simulink library "AtomicLibrary"
PostLoadFcn:
  | PacketBusGenerator; RailCabBusGenerator
(part 5 of 8)

== stateflow chart Master_Slave_Assignment_comp ==
  state chart
    state chartRegion [parallel]
      state Main
        state Synchronization [parallel]
          state Sleep
            entry: clientAvailableStatechart = true
            exit: clientAvailableStatechart = false
          state State
            entry: clientAvailableStatechart = true; masterAvailableStatechart = true
            exit: clientAvailableStatechart = false; masterAvailableStatechart = false
          state Client
          state Master
          state End
            entry: clientAvailableStatechart = true; masterAvailableStatechart = true
            exit: clientAvailableStatechart = false; masterAvailableStatechart = false
          chart.chartRegion.Main.Synchronization.Client -> End
          Master -> End
          Sleep -> chart.chartRegion.Main.Synchronization.Client : client
          State -> chart.chartRegion.Main.Synchronization.Client [order 2] : client
          End -> chart.chartRegion.Main.Synchronization.Client [order 1] : client
          State -> Master [order 1] : master
          End -> Master [order 2] : master
        state Master_Slave_Ass_Competitor [parallel]
          state Unset
            entry: startAssignmentAvailableMaster_Slave_Assignment_Competitor = true
            exit: startAssignmentAvailableMaster_Slave_Assignment_Competitor = false
          state MasterRequest
            entry: reset(c0)
          state MasterOk
          state Client
          state Inv_Error
          Unset -> chart.chartRegion.Main.Master_Slave_Ass_Competitor.Client [order 1]
          MasterRequest -> Unset [order 1] : [time(c0) > 20]
          MasterOk -> Unset
          Unset -> MasterRequest [order 2] : startAssignment
          MasterRequest -> Inv_Error [order 3] : [time(c0) > 20]
    state DataInit [parallel]
    DataInit -> DataInit
  (default) -> Sleep
  (default) -> Unset
  (default) -> Main
  (default) -> chart
  data: c0 local double =0.0; clientAvailableStatechart local boolean =false; masterAvailableStatechart local boolean =false; startAssignmentAvailableMaster_Slave_Assignment_Competitor local boolean =false; evtQueueIn function_input; param function_input; paramQueueIn function_input; event function_input; evtQueue function_output; paramQueue function_output; event function_input; evtQueue function_input; available function_output; event function_input; evtQueueIn function_input; paramQueueIn function_input; evtQueue function_output; paramQueue function_output; parameter function_output; clock function_input; logicalTime function_output; clock function_input
  events: startAssignment local EITHER_EDGE_EVENT; client local EITHER_EDGE_EVENT; master local EITHER_EDGE_EVENT
  function enqueue:
    | function [evtQueue, paramQueue] = enqueue(event, evtQueueIn, param, paramQueueIn) %eml 
    |  evtQueue = evtQueueIn; 
    |  paramQueue = paramQueueIn; 
    |  for i = 1:length(evtQueueIn) 
    |  if evtQueueIn(i) == uint8(0) 
    |  evtQueueIn(i) = event; 
    |  paramQueue(i) = param; 
    |  return 
    |  end 
    |  end
  function checkQueue:
    | function available = checkQueue(event, evtQueue) %eml 
    |  available = false; 
    |  for i = 1:length(evtQueue) 
    |      if evtQueue(i) == event 
    |          available = true;    
    |          return 
    |      end 
    |  end
  function dequeue:
    | function [evtQueue, paramQueue, parameter] = dequeue(event, evtQueueIn, paramQueueIn) %eml 
    |  evtQueue = evtQueueIn; 
    |  paramQueue = paramQueueIn; 
    |  parameter = 0; 
    |  for i = 1:length(evtQueue) 
    |  if evtQueue(i) == event 
    |  parameter = paramQueue(i); 
    |  for j = i:length(evtQueue)-1 
    |   evtQueue(j) = evtQueue(j+1); 
    |  paramQueue(j) = paramQueue(j+1); 
    |  end 
    |  evtQueue(length(evtQueue)) = 0; 
    |  paramQueue(length(paramQueue)) = 0; 
    |  return 
    |  end 
    |  end
  function time:
    | function logicalTime = time(clock) 
    |  sample = 0.01;  % the sample time of the system clock 
    |  %convert to pass units of time after last reset 
    |  logicalTime = uint32((clockSignal - clock)/sample);
  function reset:
    | function reset(clock) 
    |  %set clock variable to current time 
    |  clock = clockSignal;

== stateflow chart TestTurnTransmission/TestTurnTransmission_Statechart ==
  state chart
    state chartRegion [parallel]
      state Main
        state synchronization [parallel]
          state MyTurn
          state Initial
            entry: turnCHAvailableStatechart = true
            exit: turnCHAvailableStatechart = false
          state YourTurn
            entry: turnCHAvailableStatechart = true
            exit: turnCHAvailableStatechart = false
          Initial -> chart.chartRegion.Main.synchronization.MyTurn [order 2] : turnCH
          chart.chartRegion.Main.synchronization.YourTurn -> chart.chartRegion.Main.synchronization.MyTurn : turnCH
          chart.chartRegion.Main.synchronization.MyTurn -> chart.chartRegion.Main.synchronization.YourTurn : [turnCHAvailableTurn_transmission_partner]{send(turnCH, turn_transmission_partner)}
          Initial -> chart.chartRegion.Main.synchronization.YourTurn [order 1] : [turnCHAvailableTurn_transmission_partner]{send(turnCH, turn_transmission_partner)}
        state turn_transmission_partner [parallel]
          state Inactive
            entry: turnCHAvailableTurn_Transmission_Partner = true
            exit: turnCHAvailableTurn_Transmission_Partner = false
          state TimeOut
          state MyTurn
            entry: turnCHAvailableTurn_Transmission_Partner = true
            exit: turnCHAvailableTurn_Transmission_Partner = false
          state YourTurn
          state Inv_Error
          TimeOut -> Inactive
          chart.chartRegion.Main.turn_transmission_partner.MyTurn -> Inactive [order 2]
          chart.chartRegion.Main.turn_transmission_partner.MyTurn -> TimeOut [order 3] : [time(c0) > 20]
          chart.chartRegion.Main.turn_transmission_partner.YourTurn -> Inactive [order 3]
          chart.chartRegion.Main.turn_transmission_partner.YourTurn -> TimeOut [order 2] : [time(c0) > 20]
          Inactive -> chart.chartRegion.Main.turn_transmission_partner.YourTurn [order 1] : turnCH{[turn_transmission_partnerEvtWriteOut, turn_transmission_partnerParamWriteOut] = enqueue(EVT_TURN, turn_transmission_partnerEvtWriteOut, turn_transmission_partnerParamWriteOut)}
          chart.chartRegion.Main.turn_transmission_partner.MyTurn -> chart.chartRegion.Main.turn_transmission_partner.YourTurn [order 1] : turnCH{[turn_transmission_partnerEvtWriteOut, turn_transmission_partnerParamWriteOut] = enqueue(EVT_TURN, turn_transmission_partnerEvtWriteOut, turn_transmission_partnerParamWriteOut)}
          chart.chartRegion.Main.turn_transmission_partner.YourTurn -> chart.chartRegion.Main.turn_transmission_partner.MyTurn [order 3] : [(turnCHAvailableSynchronization) && ([checkQueue(EVT_TURN, turn_transmission_partnerEvtReadOut)])]{send(turnCH, synchronization)}
          Inactive -> chart.chartRegion.Main.turn_transmission_partner.MyTurn [order 3] : [(turnCHAvailableSynchronization) && ([checkQueue(EVT_TURN, turn_transmission_partnerEvtReadOut)])]{send(turnCH, synchronization)}
          chart.chartRegion.Main.turn_transmission_partner.MyTurn -> Inv_Error [order 4] : [time(c0) > 20]
          chart.chartRegion.Main.turn_transmission_partner.YourTurn -> Inv_Error [order 4] : [time(c0) > 20]
    state DataInit [parallel]
    DataInit -> DataInit : {turn_transmission_partnerEvtWriteOut = turn_transmission_partnerEvtWriteIn;
        | turn_transmission_partnerParamWriteOut = turn_transmission_partnerParamWriteIn;
        | turn_transmission_partnerEvtReadOut = turn_transmission_partnerEvtReadIn;
        | turn_transmission_partnerParamReadOut = turn_transmission_partnerParamReadIn;
        | }
  (default) -> Initial
  (default) -> Inactive
  (default) -> Main
  (default) -> chart
  data: EVT_TURN constant uint32 =7; c0 local double =0.0; EVT_TURN constant uint32 =7; turnCHAvailableStatechart local boolean =false; turnCHAvailableTurn_Transmission_Partner local boolean =false; evtQueueIn function_input; param function_input; paramQueueIn function_input; event function_input; evtQueue function_output; paramQueue function_output; event function_input; evtQueue function_input; available function_output; event function_input; evtQueueIn function_input; paramQueueIn function_input; evtQueue function_output; paramQueue function_output; parameter function_output; clock function_input; logicalTime function_output; clock function_input; clockSignal input; turn_transmission_partnerReadIn input; turn_transmission_partnerParamReadIn input; turn_transmission_partnerWriteIn input; turn_transmission_partnerParamWriteIn input; turn_transmission_partnerReadOut output; turn_transmission_partnerParamReadOut output; turn_transmission_partnerWriteOut output; turn_transmission_partnerParamWriteOut output
  events: turnCH local EITHER_EDGE_EVENT
  function enqueue:
    | function [evtQueue, paramQueue] = enqueue(event, evtQueueIn, param, paramQueueIn) %eml 
    |  evtQueue = evtQueueIn; 
    |  paramQueue = paramQueueIn; 
    |  for i = 1:length(evtQueueIn) 
    |  if evtQueueIn(i) == uint8(0) 
    |  evtQueueIn(i) = event; 
    |  paramQueue(i) = param; 
    |  return 
    |  end 
    |  end
  function checkQueue:
    | function available = checkQueue(event, evtQueue) %eml 
    |  available = false; 
    |  for i = 1:length(evtQueue) 
    |      if evtQueue(i) == event 
    |          available = true;    
    |          return 
    |      end 
    |  end
  function dequeue:
    | function [evtQueue, paramQueue, parameter] = dequeue(event, evtQueueIn, paramQueueIn) %eml 
    |  evtQueue = evtQueueIn; 
    |  paramQueue = paramQueueIn; 
    |  parameter = 0; 
    |  for i = 1:length(evtQueue) 
    |  if evtQueue(i) == event 
    |  parameter = paramQueue(i); 
    |  for j = i:length(evtQueue)-1 
    |   evtQueue(j) = evtQueue(j+1); 
    |  paramQueue(j) = paramQueue(j+1); 
    |  end 
    |  evtQueue(length(evtQueue)) = 0; 
    |  paramQueue(length(paramQueue)) = 0; 
    |  return 
    |  end 
    |  end
  function time:
    | function logicalTime = time(clock) 
    |  sample = 0.01;  % the sample time of the system clock 
    |  %convert to pass units of time after last reset 
    |  logicalTime = uint32((clockSignal - clock)/sample);
  function reset:
    | function reset(clock) 
    |  %set clock variable to current time 
    |  clock = clockSignal;

== stateflow chart TestRequestInformaitonUser/TestRequestInformaitonUser_Statechart ==
  state chart
    state chartRegion [parallel]
      state Main
        state Synchro [parallel]
          state NoRequest
          state Request
            entry: requestFailedAvailableStatechart = true; requestFinishedAvailableStatechart = true
            exit: requestFailedAvailableStatechart = false; requestFinishedAvailableStatechart = false
          state RequestFinished
          chart.chartRegion.Main.Synchro.Request -> NoRequest [order 1] : requestFailed
          chart.chartRegion.Main.Synchro.Request -> RequestFinished [order 2] : requestFinished
          NoRequest -> chart.chartRegion.Main.Synchro.Request : [startRequestAvailableRequest_information_user]{send(startRequest, request_information_user)}
        state request_information_user [parallel]
          state Result
            entry: startRequestAvailableRequest_Information_User = true
            exit: startRequestAvailableRequest_Information_User = false
          state Request
          Result -> chart.chartRegion.Main.request_information_user.Request : startRequest{[requestinformation_userEvtWriteOut, requestinformation_userParamWriteOut] = enqueue(EVT_REQUEST, requestinformation_userEvtWriteOut, requestinformation_userParamWriteOut)}
          chart.chartRegion.Main.request_information_user.Request -> Result [order 1] : [(requestFinishedAvailableSynchro) && ([checkQueue(EVT_VALUE, requestinformation_userEvtReadOut)])]{send(requestFinished, Synchro); reset(c0)}
          chart.chartRegion.Main.request_information_user.Request -> Result [order 1] : [(requestFailedAvailableSynchro) && (time(c0) >= 20)]{send(requestFailed, Synchro)}
    state DataInit [parallel]
    DataInit -> DataInit : {requestinformation_userEvtWriteOut = requestinformation_userEvtWriteIn;
        | requestinformation_userParamWriteOut = requestinformation_userParamWriteIn;
        | requestinformation_userEvtReadOut = requestinformation_userEvtReadIn;
        | requestinformation_userParamReadOut = requestinformation_userParamReadIn;
        | }
  (default) -> NoRequest
  (default) -> Result
  (default) -> Main
  (default) -> chart
  data: EVT_VALUE constant uint32 =9; EVT_REQUEST constant uint32 =8; c0 local double =0.0; EVT_REQUEST constant uint32 =8; EVT_VALUE constant uint32 =9; requestFailedAvailableStatechart local boolean =false; requestFinishedAvailableStatechart local boolean =false; startRequestAvailableRequest_Information_User local boolean =false; evtQueueIn function_input; param function_input; paramQueueIn function_input; event function_input; evtQueue function_output; paramQueue function_output; event function_input; evtQueue function_input; available function_output; event function_input; evtQueueIn function_input; paramQueueIn function_input; evtQueue function_output; paramQueue function_output; parameter function_output; clock function_input; logicalTime function_output; clock function_input; clockSignal input; requestinformation_userReadIn input; requestinformation_userParamReadIn input; requestinformation_userWriteIn input; requestinformation_userParamWriteIn input; requestinformation_userReadOut output; requestinformation_userParamReadOut output; requestinformation_userWriteOut output; requestinformation_userParamWriteOut output
  events: startRequest local EITHER_EDGE_EVENT; requestFinished local EITHER_EDGE_EVENT; requestFailed local EITHER_EDGE_EVENT
  function enqueue:
    | function [evtQueue, paramQueue] = enqueue(event, evtQueueIn, param, paramQueueIn) %eml 
    |  evtQueue = evtQueueIn; 
    |  paramQueue = paramQueueIn; 
    |  for i = 1:length(evtQueueIn) 
    |  if evtQueueIn(i) == uint8(0) 
    |  evtQueueIn(i) = event; 
    |  paramQueue(i) = param; 
    |  return 
    |  end 
    |  end
  function checkQueue:
    | function available = checkQueue(event, evtQueue) %eml 
    |  available = false; 
    |  for i = 1:length(evtQueue) 
    |      if evtQueue(i) == event 
    |          available = true;    
    |          return 
    |      end 
    |  end
  function dequeue:
    | function [evtQueue, paramQueue, parameter] = dequeue(event, evtQueueIn, paramQueueIn) %eml 
    |  evtQueue = evtQueueIn; 
    |  paramQueue = paramQueueIn; 
    |  parameter = 0; 
    |  for i = 1:length(evtQueue) 
    |  if evtQueue(i) == event 
    |  parameter = paramQueue(i); 
    |  for j = i:length(evtQueue)-1 
    |   evtQueue(j) = evtQueue(j+1); 
    |  paramQueue(j) = paramQueue(j+1); 
    |  end 
    |  evtQueue(length(evtQueue)) = 0; 
    |  paramQueue(length(paramQueue)) = 0; 
    |  return 
    |  end 
    |  end
  function time:
    | function logicalTime = time(clock) 
    |  sample = 0.01;  % the sample time of the system clock 
    |  %convert to pass units of time after last reset 
    |  logicalTime = uint32((clockSignal - clock)/sample);
  function reset:
    | function reset(clock) 
    |  %set clock variable to current time 
    |  clock = clockSignal;

== stateflow chart TestRequestInformationProvider/TestRequestInformationProvider_Statechart ==
  state chart
    state chartRegion [parallel]
      state Main
        state Snychro [parallel]
          state NoRequest
            entry: requestReceivedAvailableStatechart = true
            exit: requestReceivedAvailableStatechart = false
          state HandleRequest
            entry: reset(c0)
          NoRequest -> HandleRequest : requestReceived
          HandleRequest -> NoRequest : [(requestHandledAvailableRequest_information_provider) && (time(c0) >= 20)]{send(requestHandled, request_information_provider)}
        state request_information_provider [parallel]
          state Wait
          state Work
            entry: requestHandledAvailableRequest_Information_Provider = true
            exit: requestHandledAvailableRequest_Information_Provider = false
          Work -> Wait : requestHandled{[requestinformation_providerEvtWriteOut, requestinformation_providerParamWriteOut] = enqueue(EVT_VALUE, requestinformation_providerEvtWriteOut, requestinformation_providerParamWriteOut)}
          Wait -> Work : [(requestReceivedAvailableSnychro) && ([checkQueue(EVT_REQUEST, requestinformation_providerEvtReadOut)])]{send(requestReceived, Snychro)}
    state DataInit [parallel]
    DataInit -> DataInit : {requestinformation_providerEvtWriteOut = requestinformation_providerEvtWriteIn;
        | requestinformation_providerParamWriteOut = requestinformation_providerParamWriteIn;
        | requestinformation_providerEvtReadOut = requestinformation_providerEvtReadIn;
        | requestinformation_providerParamReadOut = requestinformation_providerParamReadIn;
        | }
  (default) -> NoRequest
  (default) -> Wait
  (default) -> Main
  (default) -> chart
  data: c0 local double =0.0; EVT_REQUEST constant uint32 =8; EVT_VALUE constant uint32 =9; EVT_VALUE constant uint32 =9; EVT_REQUEST constant uint32 =8; requestReceivedAvailableStatechart local boolean =false; requestHandledAvailableRequest_Information_Provider local boolean =false; evtQueueIn function_input; param function_input; paramQueueIn function_input; event function_input; evtQueue function_output; paramQueue function_output; event function_input; evtQueue function_input; available function_output; event function_input; evtQueueIn function_input; paramQueueIn function_input; evtQueue function_output; paramQueue function_output; parameter function_output; clock function_input; logicalTime function_output; clock function_input; clockSignal input; requestinformation_providerReadIn input; requestinformation_providerParamReadIn input; requestinformation_providerWriteIn input; requestinformation_providerParamWriteIn input; requestinformation_providerReadOut output; requestinformation_providerParamReadOut output; requestinformation_providerWriteOut output; requestinformation_providerParamWriteOut output
  events: requestReceived local EITHER_EDGE_EVENT; requestHandled local EITHER_EDGE_EVENT
  function enqueue:
    | function [evtQueue, paramQueue] = enqueue(event, evtQueueIn, param, paramQueueIn) %eml 
    |  evtQueue = evtQueueIn; 
    |  paramQueue = paramQueueIn; 
    |  for i = 1:length(evtQueueIn) 
    |  if evtQueueIn(i) == uint8(0) 
    |  evtQueueIn(i) = event; 
    |  paramQueue(i) = param; 
    |  return 
    |  end 
    |  end
  function checkQueue:
    | function available = checkQueue(event, evtQueue) %eml 
    |  available = false; 
    |  for i = 1:length(evtQueue) 
    |      if evtQueue(i) == event 
    |          available = true;    
    |          return 
    |      end 
    |  end
  function dequeue:
    | function [evtQueue, paramQueue, parameter] = dequeue(event, evtQueueIn, paramQueueIn) %eml 
    |  evtQueue = evtQueueIn; 
    |  paramQueue = paramQueueIn; 
    |  parameter = 0; 
    |  for i = 1:length(evtQueue) 
    |  if evtQueue(i) == event 
    |  parameter = paramQueue(i); 
    |  for j = i:length(evtQueue)-1 
    |   evtQueue(j) = evtQueue(j+1); 
    |  paramQueue(j) = paramQueue(j+1); 
    |  end 
    |  evtQueue(length(evtQueue)) = 0; 
    |  paramQueue(length(paramQueue)) = 0; 
    |  return 
    |  end 
    |  end
  function time:
    | function logicalTime = time(clock) 
    |  sample = 0.01;  % the sample time of the system clock 
    |  %convert to pass units of time after last reset 
    |  logicalTime = uint32((clockSignal - clock)/sample);
  function reset:
    | function reset(clock) 
    |  %set clock variable to current time 
    |  clock = clockSignal;

== stateflow chart TestStartStopMaster/TestStartStopMaster_Statechart ==
  state chart
    state chartRegion [parallel]
      state Main
        state Synch [parallel]
          state Initial
          state Working
          state Finished
          Initial -> Working : [startAvailableStartStop_Master]{send(start, startStop_Master); reset(c0)}
          Working -> Finished : [(finishedAvailableStartStop_Master) && (time(c0) > 20)]{send(finished, startStop_Master)}
        state startStop_Master [parallel]
          state Started
            entry: finishedAvailableStartStop_Master = true
            exit: finishedAvailableStartStop_Master = false
          state Stopped
            entry: startAvailableStartStop_Master = true
            exit: startAvailableStartStop_Master = false
          Stopped -> Started : start{[startStop_MasterEvtWriteOut, startStop_MasterParamWriteOut] = enqueue(EVT_START, startStop_MasterEvtWriteOut, startStop_MasterParamWriteOut)}
          Started -> Stopped : finished{[startStop_MasterEvtWriteOut, startStop_MasterParamWriteOut] = enqueue(EVT_STOP, startStop_MasterEvtWriteOut, startStop_MasterParamWriteOut)}
    state DataInit [parallel]
    DataInit -> DataInit : {startStop_MasterEvtWriteOut = startStop_MasterEvtWriteIn;
        | startStop_MasterParamWriteOut = startStop_MasterParamWriteIn;
        | startStop_MasterEvtReadOut = startStop_MasterEvtReadIn;
        | startStop_MasterParamReadOut = startStop_MasterParamReadIn;
        | }
  (default) -> Initial
  (default) -> Stopped
  (default) -> Main
  (default) -> chart
  data: c0 local double =0.0; EVT_START constant uint32 =10; EVT_STOP constant uint32 =11; EVT_START constant uint32 =10; EVT_STOP constant uint32 =11; startAvailableStartStop_Master local boolean =false; finishedAvailableStartStop_Master local boolean =false; evtQueueIn function_input; param function_input; paramQueueIn function_input; event function_input; evtQueue function_output; paramQueue function_output; event function_input; evtQueue function_input; available function_output; event function_input; evtQueueIn function_input; paramQueueIn function_input; evtQueue function_output; paramQueue function_output; parameter function_output; clock function_input; logicalTime function_output; clock function_input; clockSignal input; startStop_MasterReadIn input; startStop_MasterParamReadIn input; startStop_MasterWriteIn input; startStop_MasterParamWriteIn input; startStop_MasterReadOut output; startStop_MasterParamReadOut output; startStop_MasterWriteOut output; startStop_MasterParamWriteOut output
  events: start local EITHER_EDGE_EVENT; finished local EITHER_EDGE_EVENT
  function enqueue:
    | function [evtQueue, paramQueue] = enqueue(event, evtQueueIn, param, paramQueueIn) %eml 
    |  evtQueue = evtQueueIn; 
    |  paramQueue = paramQueueIn; 
    |  for i = 1:length(evtQueueIn) 
    |  if evtQueueIn(i) == uint8(0) 
    |  evtQueueIn(i) = event; 
    |  paramQueue(i) = param; 
    |  return 
    |  end 
    |  end
  function checkQueue:
    | function available = checkQueue(event, evtQueue) %eml 
    |  available = false; 
    |  for i = 1:length(evtQueue) 
    |      if evtQueue(i) == event 
    |          available = true;    
    |          return 
    |      end 
    |  end
  function dequeue:
    | function [evtQueue, paramQueue, parameter] = dequeue(event, evtQueueIn, paramQueueIn) %eml 
    |  evtQueue = evtQueueIn; 
    |  paramQueue = paramQueueIn; 
    |  parameter = 0; 
    |  for i = 1:length(evtQueue) 
    |  if evtQueue(i) == event 
    |  parameter = paramQueue(i); 
    |  for j = i:length(evtQueue)-1 
    |   evtQueue(j) = evtQueue(j+1); 
    |  paramQueue(j) = paramQueue(j+1); 
    |  end 
    |  evtQueue(length(evtQueue)) = 0; 
    |  paramQueue(length(paramQueue)) = 0; 
    |  return 
    |  end 
    |  end
  function time:
    | function logicalTime = time(clock) 
    |  sample = 0.01;  % the sample time of the system clock 
    |  %convert to pass units of time after last reset 
    |  logicalTime = uint32((clockSignal - clock)/sample);
  function reset:
    | function reset(clock) 
    |  %set clock variable to current time 
    |  clock = clockSignal;

== stateflow chart TestStartStopSlave/TestStartStopSlave_Statechart ==
  state chart
    state chartRegion [parallel]
      state Main
        state Synch [parallel]
          state Stopped
            entry: startAvailableStatechart = true
            exit: startAvailableStatechart = false
          state Working
            entry: stopAvailableStatechart = true
            exit: stopAvailableStatechart = false
          Working -> chart.chartRegion.Main.Synch.Stopped : stop
          chart.chartRegion.Main.Synch.Stopped -> Working : start
        state StartStop_Slave [parallel]
          state Stopped
          state Started
          chart.chartRegion.Main.StartStop_Slave.Stopped -> Started : [(startAvailableSynch) && ([checkQueue(EVT_START, startStop_SlaveEvtReadOut)])]{send(start, Synch)}
          Started -> chart.chartRegion.Main.StartStop_Slave.Stopped : [(stopAvailableSynch) && ([checkQueue(EVT_STOP, startStop_SlaveEvtReadOut)])]{send(stop, Synch)}
    state DataInit [parallel]
    DataInit -> DataInit : {startStop_SlaveEvtWriteOut = startStop_SlaveEvtWriteIn;
        | startStop_SlaveParamWriteOut = startStop_SlaveParamWriteIn;
        | startStop_SlaveEvtReadOut = startStop_SlaveEvtReadIn;
        | startStop_SlaveParamReadOut = startStop_SlaveParamReadIn;
        | }
  (default) -> chart.chartRegion.Main.Synch.Stopped
  (default) -> chart.chartRegion.Main.StartStop_Slave.Stopped
  (default) -> Main
  (default) -> chart
  data: EVT_START constant uint32 =10; EVT_STOP constant uint32 =11; EVT_START constant uint32 =10; EVT_STOP constant uint32 =11; stopAvailableStatechart local boolean =false; startAvailableStatechart local boolean =false; evtQueueIn function_input; param function_input; paramQueueIn function_input; event function_input; evtQueue function_output; paramQueue function_output; event function_input; evtQueue function_input; available function_output; event function_input; evtQueueIn function_input; paramQueueIn function_input; evtQueue function_output; paramQueue function_output; parameter function_output; clock function_input; logicalTime function_output; clock function_input; clockSignal input; startStop_SlaveReadIn input; startStop_SlaveParamReadIn input; startStop_SlaveWriteIn input; startStop_SlaveParamWriteIn input; startStop_SlaveReadOut output; startStop_SlaveParamReadOut output; startStop_SlaveWriteOut output; startStop_SlaveParamWriteOut output
  events: stop local EITHER_EDGE_EVENT; start local EITHER_EDGE_EVENT
  function enqueue:
    | function [evtQueue, paramQueue] = enqueue(event, evtQueueIn, param, paramQueueIn) %eml 
    |  evtQueue = evtQueueIn; 
    |  paramQueue = paramQueueIn; 
    |  for i = 1:length(evtQueueIn) 
    |  if evtQueueIn(i) == uint8(0) 
    |  evtQueueIn(i) = event; 
    |  paramQueue(i) = param; 
    |  return 
    |  end 
    |  end
  function checkQueue:
    | function available = checkQueue(event, evtQueue) %eml 
    |  available = false; 
    |  for i = 1:length(evtQueue) 
    |      if evtQueue(i) == event 
    |          available = true;    
    |          return 
    |      end 
    |  end
  function dequeue:
    | function [evtQueue, paramQueue, parameter] = dequeue(event, evtQueueIn, paramQueueIn) %eml 
    |  evtQueue = evtQueueIn; 
    |  paramQueue = paramQueueIn; 
    |  parameter = 0; 
    |  for i = 1:length(evtQueue) 
    |  if evtQueue(i) == event 
    |  parameter = paramQueue(i); 
    |  for j = i:length(evtQueue)-1 
    |   evtQueue(j) = evtQueue(j+1); 
    |  paramQueue(j) = paramQueue(j+1); 
    |  end 
    |  evtQueue(length(evtQueue)) = 0; 
    |  paramQueue(length(paramQueue)) = 0; 
    |  return 
    |  end 
    |  end
  function time:
    | function logicalTime = time(clock) 
    |  sample = 0.01;  % the sample time of the system clock 
    |  %convert to pass units of time after last reset 
    |  logicalTime = uint32((clockSignal - clock)/sample);
  function reset:
    | function reset(clock) 
    |  %set clock variable to current time 
    |  clock = clockSignal;

== stateflow chart Handshake_Partner ==
  state chart
    state chartRegion [parallel]
      state Handshake_Main
    state DataInit [parallel]
    DataInit -> DataInit
  (default) -> Handshake_Main
  (default) -> chart
  data: evtQueueIn function_input; param function_input; paramQueueIn function_input; event function_input; evtQueue function_output; paramQueue function_output; event function_input; evtQueue function_input; available function_output; event function_input; evtQueueIn function_input; paramQueueIn function_input; evtQueue function_output; paramQueue function_output; parameter function_output; clock function_input; logicalTime function_output; clock function_input
  function enqueue:
    | function [evtQueue, paramQueue] = enqueue(event, evtQueueIn, param, paramQueueIn) %eml 
    |  evtQueue = evtQueueIn; 
    |  paramQueue = paramQueueIn; 
    |  for i = 1:length(evtQueueIn) 
    |  if evtQueueIn(i) == uint8(0) 
    |  evtQueueIn(i) = event; 
    |  paramQueue(i) = param; 
    |  return 
    |  end 
    |  end
  function checkQueue:
    | function available = checkQueue(event, evtQueue) %eml 
    |  available = false; 
    |  for i = 1:length(evtQueue) 
    |      if evtQueue(i) == event 
    |          available = true;    
    |          return 
    |      end 
    |  end
  function dequeue:
    | function [evtQueue, paramQueue, parameter] = dequeue(event, evtQueueIn, paramQueueIn) %eml 
    |  evtQueue = evtQueueIn; 
    |  paramQueue = paramQueueIn; 
    |  parameter = 0; 
    |  for i = 1:length(evtQueue) 
    |  if evtQueue(i) == event 
    |  parameter = paramQueue(i); 
    |  for j = i:length(evtQueue)-1 
    |   evtQueue(j) = evtQueue(j+1); 
    |  paramQueue(j) = paramQueue(j+1); 
    |  end 
    |  evtQueue(length(evtQueue)) = 0; 
    |  paramQueue(length(paramQueue)) = 0; 
    |  return 
    |  end 
    |  end
  function time:
    | function logicalTime = time(clock) 
    |  sample = 0.01;  % the sample time of the system clock 
    |  %convert to pass units of time after last reset 
    |  logicalTime = uint32((clockSignal - clock)/sample);
  function reset:
    | function reset(clock) 
    |  %set clock variable to current time 
    |  clock = clockSignal;

== stateflow chart  ==
  state chart
    state chartRegion [parallel]
      state Main
        state synch [parallel]
        state Handshake.Partner [parallel]
    state DataInit [parallel]
    DataInit -> DataInit
  (default) -> Main
  (default) -> chart
  data: evtQueueIn function_input; param function_input; paramQueueIn function_input; event function_input; evtQueue function_output; paramQueue function_output; event function_input; evtQueue function_input; available function_output; event function_input; evtQueueIn function_input; paramQueueIn function_input; evtQueue function_output; paramQueue function_output; parameter function_output; clock function_input; logicalTime function_output; clock function_input
  function enqueue:
    | function [evtQueue, paramQueue] = enqueue(event, evtQueueIn, param, paramQueueIn) %eml 
    |  evtQueue = evtQueueIn; 
    |  paramQueue = paramQueueIn; 
    |  for i = 1:length(evtQueueIn) 
    |  if evtQueueIn(i) == uint8(0) 
    |  evtQueueIn(i) = event; 
    |  paramQueue(i) = param; 
    |  return 
    |  end 
    |  end
  function checkQueue:
    | function available = checkQueue(event, evtQueue) %eml 
    |  available = false; 
    |  for i = 1:length(evtQueue) 
    |      if evtQueue(i) == event 
    |          available = true;    
    |          return 
    |      end 
    |  end
  function dequeue:
    | function [evtQueue, paramQueue, parameter] = dequeue(event, evtQueueIn, paramQueueIn) %eml 
    |  evtQueue = evtQueueIn; 
    |  paramQueue = paramQueueIn; 
    |  parameter = 0; 
    |  for i = 1:length(evtQueue) 
    |  if evtQueue(i) == event 
    |  parameter = paramQueue(i); 
    |  for j = i:length(evtQueue)-1 
    |   evtQueue(j) = evtQueue(j+1); 
    |  paramQueue(j) = paramQueue(j+1); 
    |  end 
    |  evtQueue(length(evtQueue)) = 0; 
    |  paramQueue(length(paramQueue)) = 0; 
    |  return 
    |  end 
    |  end
  function time:
    | function logicalTime = time(clock) 
    |  sample = 0.01;  % the sample time of the system clock 
    |  %convert to pass units of time after last reset 
    |  logicalTime = uint32((clockSignal - clock)/sample);
  function reset:
    | function reset(clock) 
    |  %set clock variable to current time 
    |  clock = clockSignal;

== stateflow chart Pattern_Delegation_Slave ==
  state chart
    state chartRegion [parallel]
      state Inactive
      state Success
      state Fail
      state Running
    state DataInit [parallel]
    DataInit -> DataInit
  (default) -> chart
  data: evtQueueIn function_input; param function_input; paramQueueIn function_input; event function_input; evtQueue function_output; paramQueue function_output; event function_input; evtQueue function_input; available function_output; event function_input; evtQueueIn function_input; paramQueueIn function_input; evtQueue function_output; paramQueue function_output; parameter function_output; clock function_input; logicalTime function_output; clock function_input
  function enqueue:
    | function [evtQueue, paramQueue] = enqueue(event, evtQueueIn, param, paramQueueIn) %eml 
    |  evtQueue = evtQueueIn; 
    |  paramQueue = paramQueueIn; 
    |  for i = 1:length(evtQueueIn) 
    |  if evtQueueIn(i) == uint8(0) 
    |  evtQueueIn(i) = event; 
    |  paramQueue(i) = param; 
    |  return 
    |  end 
    |  end
  function checkQueue:
    | function available = checkQueue(event, evtQueue) %eml 
    |  available = false; 
    |  for i = 1:length(evtQueue) 
    |      if evtQueue(i) == event 
    |          available = true;    
    |          return 
    |      end 
    |  end
  function dequeue:
    | function [evtQueue, paramQueue, parameter] = dequeue(event, evtQueueIn, paramQueueIn) %eml 
    |  evtQueue = evtQueueIn; 
    |  paramQueue = paramQueueIn; 
    |  parameter = 0; 
    |  for i = 1:length(evtQueue) 
    |  if evtQueue(i) == event 
    |  parameter = paramQueue(i); 
    |  for j = i:length(evtQueue)-1 
    |   evtQueue(j) = evtQueue(j+1); 
    |  paramQueue(j) = paramQueue(j+1); 
    |  end 
    |  evtQueue(length(evtQueue)) = 0; 
    |  paramQueue(length(paramQueue)) = 0; 
    |  return 
    |  end 
    |  end
  function time:
    | function logicalTime = time(clock) 
    |  sample = 0.01;  % the sample time of the system clock 
    |  %convert to pass units of time after last reset 
    |  logicalTime = uint32((clockSignal - clock)/sample);
  function reset:
    | function reset(clock) 
    |  %set clock variable to current time 
    |  clock = clockSignal;

== stateflow chart Pattern_EventListener_Master ==
  state chart
    state chartRegion [parallel]
      state State
      State -> State
    state DataInit [parallel]
    DataInit -> DataInit
  (default) -> State
  (default) -> chart
  data: evtQueueIn function_input; param function_input; paramQueueIn function_input; event function_input; evtQueue function_output; paramQueue function_output; event function_input; evtQueue function_input; available function_output; event function_input; evtQueueIn function_input; paramQueueIn function_input; evtQueue function_output; paramQueue function_output; parameter function_output; clock function_input; logicalTime function_output; clock function_input
  function enqueue:
    | function [evtQueue, paramQueue] = enqueue(event, evtQueueIn, param, paramQueueIn) %eml 
    |  evtQueue = evtQueueIn; 
    |  paramQueue = paramQueueIn; 
    |  for i = 1:length(evtQueueIn) 
    |  if evtQueueIn(i) == uint8(0) 
    |  evtQueueIn(i) = event; 
    |  paramQueue(i) = param; 
    |  return 
    |  end 
    |  end
  function checkQueue:
    | function available = checkQueue(event, evtQueue) %eml 
    |  available = false; 
    |  for i = 1:length(evtQueue) 
    |      if evtQueue(i) == event 
    |          available = true;    
    |          return 
    |      end 
    |  end
  function dequeue:
    | function [evtQueue, paramQueue, parameter] = dequeue(event, evtQueueIn, paramQueueIn) %eml 
    |  evtQueue = evtQueueIn; 
    |  paramQueue = paramQueueIn; 
    |  parameter = 0; 
    |  for i = 1:length(evtQueue) 
    |  if evtQueue(i) == event 
    |  parameter = paramQueue(i); 
    |  for j = i:length(evtQueue)-1 
    |   evtQueue(j) = evtQueue(j+1); 
    |  paramQueue(j) = paramQueue(j+1); 
    |  end 
    |  evtQueue(length(evtQueue)) = 0; 
    |  paramQueue(length(paramQueue)) = 0; 
    |  return 
    |  end 
    |  end
  function time:
    | function logicalTime = time(clock) 
    |  sample = 0.01;  % the sample time of the system clock 
    |  %convert to pass units of time after last reset 
    |  logicalTime = uint32((clockSignal - clock)/sample);
  function reset:
    | function reset(clock) 
    |  %set clock variable to current time 
    |  clock = clockSignal;

== stateflow chart UserInterface/UserInterface_Statechart ==
  state chart
    state chartRegion [parallel]
      state Main
    state DataInit [parallel]
    DataInit -> DataInit : {HMI_STRATEGYREQUEST.providerEvtWriteOut = HMI_STRATEGYREQUEST.providerEvtWriteIn;
        | HMI_STRATEGYREQUEST.providerParamWriteOut = HMI_STRATEGYREQUEST.providerParamWriteIn;
        | HMI_STRATEGYREQUEST.providerEvtReadOut = HMI_STRATEGYREQUEST.providerEvtReadIn;
        | HMI_STRATEGYREQUEST.providerParamReadOut = HMI_STRATEGYREQUEST.providerParamReadIn;
        | HMI_RESET.masterEvtWriteOut = HMI_RESET.masterEvtWriteIn;
        | HMI_RESET.masterParamWriteOut = HMI_RESET.masterParamWriteIn;
        | HMI_RESET.masterEvtReadOut = HMI_RESET.masterEvtReadIn;
        | HMI_RESET.masterParamReadOut = HMI_RESET.masterParamReadIn;
        | HMI_STRATEGY.masterEvtWriteOut = HMI_STRATEGY.masterEvtWriteIn;
        | HMI_STRATEGY.masterParamWriteOut = HMI_STRATEGY.masterParamWriteIn;
        | HMI_STRATEGY.masterEvtReadOut = HMI_STRATEGY.masterEvtReadIn;
        | HMI_STRATEGY.masterParamReadOut = HMI_STRATEGY.masterParamReadIn;
        | STATUS.slaveEvtWriteOut = STATUS.slaveEvtWriteIn;
        | STATUS.slaveParamWriteOut = STATUS.slaveParamWriteIn;
        | STATUS.slaveEvtReadOut = STATUS.slaveEvtReadIn;
        | STATUS.slaveParamReadOut = STATUS.slaveParamReadIn;
        | HMI_END.masterEvtWriteOut = HMI_END.masterEvtWriteIn;
        | HMI_END.masterParamWriteOut = HMI_END.masterParamWriteIn;
        | HMI_END.masterEvtReadOut = HMI_END.masterEvtReadIn;
        | HMI_END.masterParamReadOut = HMI_END.masterParamReadIn;
        | }
  (default) -> Main
  (default) -> chart
  data: evtQueueIn function_input; param function_input; paramQueueIn function_input; event function_input; evtQueue function_output; paramQueue function_output; event function_input; evtQueue function_input; available function_output; event function_input; evtQueueIn function_input; paramQueueIn function_input; evtQueue function_output; paramQueue function_output; parameter function_output; clock function_input; logicalTime function_output; clock function_input; clockSignal input; HMI_STRATEGYREQUEST.providerReadIn input; HMI_STRATEGYREQUEST.providerParamReadIn input; HMI_STRATEGYREQUEST.providerWriteIn input; HMI_STRATEGYREQUEST.providerParamWriteIn input; HMI_RESET.masterReadIn input; HMI_RESET.masterParamReadIn input; HMI_RESET.masterWriteIn input; HMI_RESET.masterParamWriteIn input; HMI_STRATEGY.masterReadIn input; HMI_STRATEGY.masterParamReadIn input; HMI_STRATEGY.masterWriteIn input; HMI_STRATEGY.masterParamWriteIn input; STATUS.slaveReadIn input; STATUS.slaveParamReadIn input; STATUS.slaveWriteIn input; STATUS.slaveParamWriteIn input; HMI_END.masterReadIn input; HMI_END.masterParamReadIn input; HMI_END.masterWriteIn input; HMI_END.masterParamWriteIn input; HMI_STRATEGYREQUEST.providerReadOut output; HMI_STRATEGYREQUEST.providerParamReadOut output; HMI_STRATEGYREQUEST.providerWriteOut output; HMI_STRATEGYREQUEST.providerParamWriteOut output; HMI_RESET.masterReadOut output; HMI_RESET.masterParamReadOut output; HMI_RESET.masterWriteOut output; HMI_RESET.masterParamWriteOut output; HMI_STRATEGY.masterReadOut output; HMI_STRATEGY.masterParamReadOut output; HMI_STRATEGY.masterWriteOut output; HMI_STRATEGY.masterParamWriteOut output; STATUS.slaveReadOut output; STATUS.slaveParamReadOut output; STATUS.slaveWriteOut output; STATUS.slaveParamWriteOut output; HMI_END.masterReadOut output; HMI_END.masterParamReadOut output; HMI_END.masterWriteOut output; HMI_END.masterParamWriteOut output
  function enqueue:
    | function [evtQueue, paramQueue] = enqueue(event, evtQueueIn, param, paramQueueIn) %eml 
    |  evtQueue = evtQueueIn; 
    |  paramQueue = paramQueueIn; 
    |  for i = 1:length(evtQueueIn) 
    |  if evtQueueIn(i) == uint8(0) 
    |  evtQueueIn(i) = event; 
    |  paramQueue(i) = param; 
    |  return 
    |  end 
    |  end
  function checkQueue:
    | function available = checkQueue(event, evtQueue) %eml 
    |  available = false; 
    |  for i = 1:length(evtQueue) 
    |      if evtQueue(i) == event 
    |          available = true;    
    |          return 
    |      end 
    |  end
  function dequeue:
    | function [evtQueue, paramQueue, parameter] = dequeue(event, evtQueueIn, paramQueueIn) %eml 
    |  evtQueue = evtQueueIn; 
    |  paramQueue = paramQueueIn; 
    |  parameter = 0; 
    |  for i = 1:length(evtQueue) 
    |  if evtQueue(i) == event 
    |  parameter = paramQueue(i); 
    |  for j = i:length(evtQueue)-1 
    |   evtQueue(j) = evtQueue(j+1); 
    |  paramQueue(j) = paramQueue(j+1); 
    |  end 
    |  evtQueue(length(evtQueue)) = 0; 
    |  paramQueue(length(paramQueue)) = 0; 
    |  return 
    |  end 
    |  end
  function time:
    | function logicalTime = time(clock) 
    |  sample = 0.01;  % the sample time of the system clock 
    |  %convert to pass units of time after last reset 
    |  logicalTime = uint32((clockSignal - clock)/sample);
  function reset:
    | function reset(clock) 
    |  %set clock variable to current time 
    |  clock = clockSignal;

== matlab function UserInterface/Link Layer HMI_STRATEGYREQUEST.provider/DataLinkLayer/Embedded MATLAB Function ==
  data: snd_from_in input; snd_to_in input; snd_msg_in input; snd_param_in input; recv_from_in input; recv_to_in input; recv_msg_in input; recv_param_in input; recv_pkgid_in input uint32; recv_time_in input; currentTime input; from output; to output; msg output; param output; pkgid output; recv_from_out output; recv_msg_out output; recv_param_out output; time output; queue_sending_ratio output; queue_received_ratio output; queue_ack_ratio output
function [from, to, msg, param, pkgid, recv_from_out, recv_msg_out, recv_param_out, time, queue_sending_ratio, queue_received_ratio, queue_ack_ratio] = ackHandler(snd_from_in, snd_to_in, snd_msg_in, snd_param_in, recv_from_in, recv_to_in, recv_msg_in, recv_param_in, recv_pkgid_in, recv_time_in, currentTime)
%#eml
eml.extrinsic('warning', 'disp', 'fprintf');

%Constants
BUS_SIZE =  numel(snd_msg_in);
TIMEOUT_ACK     = 2.0;
MSG_ACK         = 255;
QUEUE_SIZE_SENDING = 10 * BUS_SIZE;
QUEUE_SIZE_ACK  = 10* BUS_SIZE;
QUEUE_SIZE_RECEIVED = 10 *BUS_SIZE;


%Init
from    = zeros(1,BUS_SIZE,'uint8');
to      = zeros(1,BUS_SIZE,'uint8');
msg     = zeros(1,BUS_SIZE,'uint16');
param   = zeros(1,BUS_SIZE,'double');
pkgid   = zeros(1,BUS_SIZE,'uint32');
time    = zeros(1,BUS_SIZE,'double');
 
recv_from_out    = zeros(1,BUS_SIZE,'uint8');
recv_msg_out     = zeros(1,BUS_SIZE,'uint16');
recv_param_out   = zeros(1,BUS_SIZE,'double');


recv_in = bus(recv_from_in, recv_to_in, recv_msg_in, recv_param_in, recv_pkgid_in, recv_time_in, BUS_SIZE);



%Persistent variables
persistent sendingQueue ackQueue receivedQueue lastPkgid

if isempty(lastPkgid)
    lastPkgid = uint32(0);
end

if isempty(sendingQueue)
    sendingQueue = repmat(packet(0,0,0,0,0,0), 1, QUEUE_SIZE_SENDING);
end

if isempty(ackQueue)
    ackQueue = repmat(packet(0,0,0,0,0,0), 1, QUEUE_SIZE_ACK);
end

if isempty(receivedQueue)
    receivedQueue = repmat(packet(0, 0, 0, 0, 0, 0), 1, QUEUE_SIZE_RECEIVED);
end

%compute stats
queue_sending_ratio = queueNumElements(sendingQueue)/QUEUE_SIZE_SENDING;
queue_ack_ratio = queueNumElements(ackQueue)/QUEUE_SIZE_ACK;
queue_received_ratio = queueNumElements(receivedQueue)/QUEUE_SIZE_RECEIVED;

%Step 1: Check for a new outgoing packet
for i = 1:BUS_SIZE    
    if snd_msg_in(i) ~= 0
        lastPkgid = lastPkgid +1;
        outgoing = packet(snd_from_in, snd_to_in, snd_msg_in(i), snd_param_in(i), lastPkgid, currentTime);

        %Add packet so the outgoing queue
        sendingQueue = enqueue(sendingQueue, outgoing); 
    end
end
    
%Step 2: Check for a new incoming packet
for i = 1:length(recv_in)
    incoming = packet(recv_in(i).from, recv_in(i).to, recv_in(i).msg, recv_in(i).param, recv_in(i).pkgid, recv_in(i).time);
    if incoming.from ~= 0 && incoming.to == snd_from_in
        if incoming.msg == MSG_ACK
            %Remove packet from ackQueue
            for j=1:length(ackQueue)
                if ackQueue(j).pkgid == uint32(incoming.param)
                    ackQueue = dequeue(ackQueue,j);
                    break;
                end
            end
        else
            %Send ACK
            ackPacket = packet(incoming.to, incoming.from, MSG_ACK, double(incoming.pkgid),incoming.pkgid, currentTime);
            sendingQueue = enqueue(sendingQueue,ackPacket);

            %Check for duplicated packets
            duplicatedPacket = false;
            for j=1:length(receivedQueue)
                if receivedQueue(j).pkgid == incoming.pkgid && receivedQueue(j).from == incoming.from
                    duplicatedPacket = true;
                    break;
                end
            end

            if duplicatedPacket == false
                %save packet
                receivedQueue = enqueue(receivedQueue, incoming);            
            end
        end
    end
end

%Step 3: Forward incoming packet
for i = 1:BUS_SIZE
    if receivedQueue(1).from ~= 0
        recv_from_out(i)    = receivedQueue(1).from;
        recv_msg_out(i)     = receivedQueue(1).msg;
        recv_param_out(i)   = receivedQueue(1).param;
        receivedQueue = dequeue(receivedQueue,1);
    else
        break;
    end
end

%Step 4: Timeout reached? Send packet again
for i = 1:length(ackQueue)
    if ackQueue(i).to ~= 0
        if ackQueue(i).time + TIMEOUT_ACK <= currentTime
            %Reset counter
            ackQueue(i).time = currentTime;
            %Send again
            sendingQueue = enqueue(sendingQueue, ackQueue(i));
            %Remove packet from ackQueue
            ackQueue = dequeue(ackQueue, i);
        end
    end
end


%Step 5: Send outgoing packet
for i = 1:BUS_SIZE
    if sendingQueue(1).to ~= 0    
        from(i)    = sendingQueue(1).from;
        to(i)      = sendingQueue(1).to;
        msg(i)     = sendingQueue(1).msg;
        param(i)   = sendingQueue(1).param;
        pkgid(i)   = sendingQueue(1).pkgid;
        time(i)    = sendingQueue(1).time;

        %Add it to the ack queue
        if sendingQueue(1).msg ~= MSG_ACK
            ackQueue = enqueue(ackQueue, sendingQueue(1));
        end

        %remove packet from sending queue
        sendingQueue = dequeue(sendingQueue, 1);    
    else
        break;
    end
end


%%%%%%%%%%%%%%%%%%%%%%%%%%%%%%%%%%%%%%%%%%%%%%%%%%%%%%%%%%%%%%%%%%%%%%%%%%%
%%                          H E L P E R
%%%%%%%%%%%%%%%%%%%%%%%%%%%%%%%%%%%%%%%%%%%%%%%%%%%%%%%%%%%%%%%%%%%%%%%%%%%

function p = packet(from, to, msg, param, pkgid, time)
%#eml
%Defines a packet
p = struct('from', uint8(from),'to', uint8(to),'msg', uint16(msg),'param', double(param),'pkgid', uint32(pkgid), 'time', double(time));

function bus = bus(from, to, msg, param, pkgid, time, size) %emp
%Create an empty bus
bus = repmat(packet(0,0,0,0,0,0), 1, size);
for i=1:size
    bus(i) = packet(from(i), to(i), msg(i), param(i), pkgid(i), time(i));
end


function queue = enqueue(queue, packet)
%#eml
eml.extrinsic('warning', 'sprintf');
for i = 1:length(queue)
    if queue(i).to == 0
        queue(i) = packet;
        return;
    end
end
warning('RailCab:DataLinkLayer', 'DataLinkLayer Buffer overflow. Dropping packet  %3u: %u->%u :%3u (%.1f) @%.2f', packet.pkgid, packet.from, packet.to, packet.msg, packet.param, packet.time);

function queue = dequeue(queue, index)
%#eml
assert(index <= length(queue))
for i=index:length(queue)-1;
    queue(i) = queue(i+1);
end
queue(length(queue)) = packet(0,0,0,0,0,0);

function num = queueNumElements(queue)
%#eml
num = 0;
for i = 1:length(queue)
    if queue(i).to ~= uint8(0)
        num = num+1;
    end
end    

function packetString = toString(packet) %#eml
eml.extrinsic('sprintf');
packetString = sprintf('%3u: %u->%u :%3u (%.1f) @%.2f', packet.pkgid, packet.from, packet.to, packet.msg, packet.param, packet.time);
